simulink model "exp11_5"  (R2020a)
settings: Solver=FixedStepAuto  StartTime=0.0  StopTime=5  FixedStep=0.01  RelTol=1e-3
libraries: fl_lib x39, nesl_utility x3
settings Model: Creator=Sing Ngai  LastModifiedBy=zengw

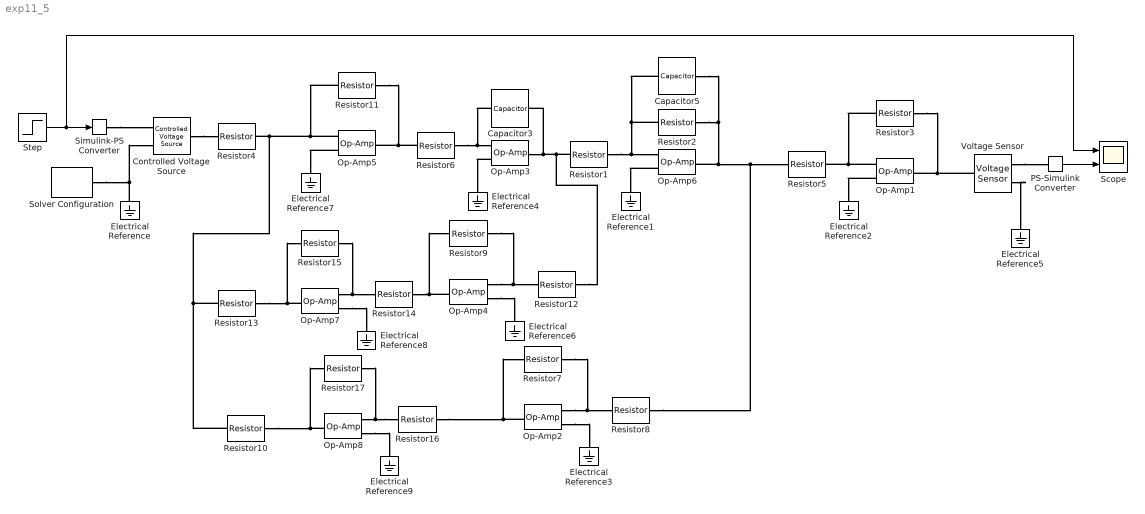
== system exp11_5 ==
  Capacitor3 : fl_lib/Electrical/Electrical Elements/Capacitor  c=2 uF  r=1e-6 Ohm  g=0 1/Ohm  i_specify=off  i_priority=None  i=0 A  i_nominal_specify=off  i_nominal_unit=A  i_nominal_value=1  v_specify=off  v_priority=None  v=0 V  v_nominal_specify=off  v_nominal_unit=V  v_nominal_value=1  vc_specify=off  vc_priority=High  vc=0 V  vc_nominal_specify=off  vc_nominal_unit=V  vc_nominal_value=1
  Capacitor5 : fl_lib/Electrical/Electrical Elements/Capacitor  c=1 uF  r=1e-6 Ohm  g=0 1/Ohm  i_specify=off  i_priority=None  i=0 A  i_nominal_specify=off  i_nominal_unit=A  i_nominal_value=1  v_specify=off  v_priority=None  v=0 V  v_nominal_specify=off  v_nominal_unit=V  v_nominal_value=1  vc_specify=off  vc_priority=High  vc=0 V  vc_nominal_specify=off  vc_nominal_unit=V  vc_nominal_value=1
  Controlled Voltage Source : fl_lib/Electrical/Electrical Sources/Controlled Voltage Source
  Electrical Reference{,1..9} (10 alike) : fl_lib/Electrical/Electrical Elements/Electrical Reference
  Op-Amp{1..8} (8 alike) : fl_lib/Electrical/Electrical Elements/Op-Amp  outI_specify=off  outI_priority=None  outI=0 A  outI_nominal_specify=off  outI_nominal_unit=A  outI_nominal_value=1
  PS-Simulink Converter : nesl_utility/PS-Simulink Converter  PhysicalDomain=network_engine_domain  SubClassName=ps_output  LeftPortType=input  RightPortType=output  PseudoPeriodic=off  Frequencies=[]  Unit=inherit  AffineConversion=off
  Resistor1 : fl_lib/Electrical/Electrical Elements/Resistor  R=50 kOhm  i_specify=off  i_priority=None  i=0 A  i_nominal_specify=off  i_nominal_unit=A  i_nominal_value=1  v_specify=off  v_priority=None  v=0 V  v_nominal_specify=off  v_nominal_unit=V  v_nominal_value=1
  Resistor{4,10..11,13} (4 alike) : fl_lib/Electrical/Electrical Elements/Resistor  R=200 kOhm  i_specify=off  i_priority=None  i=0 A  i_nominal_specify=off  i_nominal_unit=A  i_nominal_value=1  v_specify=off  v_priority=None  v=0 V  v_nominal_specify=off  v_nominal_unit=V  v_nominal_value=1
  Resistor{3,8,12,14..17} (7 alike) : fl_lib/Electrical/Electrical Elements/Resistor  R=100 kOhm  i_specify=off  i_priority=None  i=0 A  i_nominal_specify=off  i_nominal_unit=A  i_nominal_value=1  v_specify=off  v_priority=None  v=0 V  v_nominal_specify=off  v_nominal_unit=V  v_nominal_value=1
  Resistor2 : fl_lib/Electrical/Electrical Elements/Resistor  R=50 kOhm  i_specify=off  i_priority=None  i=0 A  i_nominal_specify=off  i_nominal_unit=A  i_nominal_value=1  v_specify=off  v_priority=None  v=0 V  v_nominal_specify=off  v_nominal_unit=V  v_nominal_value=1
  Resistor5 : fl_lib/Electrical/Electrical Elements/Resistor  R=20 kOhm  i_specify=off  i_priority=None  i=0 A  i_nominal_specify=off  i_nominal_unit=A  i_nominal_value=1  v_specify=off  v_priority=None  v=0 V  v_nominal_specify=off  v_nominal_unit=V  v_nominal_value=1
  Resistor6 : fl_lib/Electrical/Electrical Elements/Resistor  R=500 kOhm  i_specify=off  i_priority=None  i=0 A  i_nominal_specify=off  i_nominal_unit=A  i_nominal_value=1  v_specify=off  v_priority=None  v=0 V  v_nominal_specify=off  v_nominal_unit=V  v_nominal_value=1
  Resistor7 : fl_lib/Electrical/Electrical Elements/Resistor  R=1300 kOhm  i_specify=off  i_priority=None  i=0 A  i_nominal_specify=off  i_nominal_unit=A  i_nominal_value=1  v_specify=off  v_priority=None  v=0 V  v_nominal_specify=off  v_nominal_unit=V  v_nominal_value=1
  Resistor9 : fl_lib/Electrical/Electrical Elements/Resistor  R=800 kOhm  i_specify=off  i_priority=None  i=0 A  i_nominal_specify=off  i_nominal_unit=A  i_nominal_value=1  v_specify=off  v_priority=None  v=0 V  v_nominal_specify=off  v_nominal_unit=V  v_nominal_value=1
  Scope : Scope  NumInputPorts=2
  Simulink-PS Converter : nesl_utility/Simulink-PS Converter  PhysicalDomain=network_engine_domain  SubClassName=ps_input  LeftPortType=input  RightPortType=output  PseudoPeriodic=off  Frequencies=[]  NoiseDistribution=none  NoiseParameters=[]  Unit=1  AffineConversion=off  FilteringAndDerivatives=provide  SimscapeFilterOrder=1  InputFilterTimeConstant=0.001  UdotUserProvided=0
  Solver Configuration : nesl_utility/Solver Configuration  PhysicalDomain=network_engine_domain  SubClassName=solver  LeftPortType=input  RightPortType=generic  Tones=[]  Harmonics=[]  SimulateNoise=off  Profile=off  UseLocalSampling=off  EnableSwitchedLinearOptims=on  FrequencyDomain=off  UseCCode=off  RelTol=0.001  AbsTol=1e-06  MinStep=1e-09  ToWorkspace=off  RevertToSquareIcSolve=off  NumHomotopyIterations=100  PhasorMode=off  PhasorModeNumHarmonics=1  DoDC=off  ResidualTolerance=1e-09  UseLocalSolver=off  LocalSolverChoice=NE_BACKWARD_EULER_ADVANCER  LocalSolverSampleTime=0.001  DoFixedCost=off  MaxNonlinIter=3  MaxModeIter=2  LinearAlgebra=auto  EquationFormulation=NE_TIME_EF  DelaysMemoryBudget=1024  AutomaticFiltering=on  FilteringTimeConstant=0.001  PartitionStorageMethod=AS_NEEDED  PartitionMemoryBudget=1024  PartitionMethod=ROBUST
  Step : Step  Before=1  SampleTime=0
  Voltage Sensor : fl_lib/Electrical/Electrical Sensors/Voltage Sensor
  wires:
  Step/1 -> Scope/1, Simulink-PS Converter/1
  PS-Simulink Converter/1 -> Scope/2
  connections:
  Op-Amp6/RConn1 -- Resistor8/LConn1 -- Resistor5/LConn1 -- Capacitor5/RConn1 -- Resistor2/RConn1
  Solver Configuration/RConn1 -- Controlled Voltage Source/RConn2 -- Electrical Reference/LConn1
  Resistor1/RConn1 -- Op-Amp6/LConn2 -- Capacitor5/LConn1 -- Resistor2/LConn1
  Op-Amp7/RConn1 -- Resistor13/LConn1 -- Resistor15/RConn1
  Op-Amp1/LConn2 -- Resistor5/RConn1 -- Resistor3/LConn1
  Op-Amp5/RConn1 -- Resistor6/LConn1 -- Resistor11/RConn1
  Op-Amp1/RConn1 -- Voltage Sensor/LConn1 -- Resistor3/RConn1
  Capacitor3/LConn1 -- Op-Amp3/LConn2 -- Resistor6/RConn1
  Op-Amp3/RConn1 -- Resistor12/LConn1 -- Resistor1/LConn1 -- Capacitor3/RConn1
  Voltage Sensor/RConn2 -- Electrical Reference5/LConn1
  Voltage Sensor/RConn1 -- PS-Simulink Converter/LConn1
  Op-Amp5/LConn1 -- Electrical Reference7/LConn1
  Op-Amp1/LConn1 -- Electrical Reference2/LConn1
  Simulink-PS Converter/RConn1 -- Controlled Voltage Source/RConn1
  Op-Amp6/LConn1 -- Electrical Reference1/LConn1
  Controlled Voltage Source/LConn1 -- Resistor4/LConn1
  Op-Amp3/LConn1 -- Electrical Reference4/LConn1
  Op-Amp2/LConn2 -- Resistor8/RConn1 -- Resistor7/LConn1
  Op-Amp2/LConn1 -- Electrical Reference3/LConn1
  Op-Amp2/RConn1 -- Resistor7/RConn1 -- Resistor16/LConn1
  Op-Amp4/LConn2 -- Resistor12/RConn1 -- Resistor9/LConn1
  Op-Amp4/RConn1 -- Resistor14/LConn1 -- Resistor9/RConn1
  Op-Amp4/LConn1 -- Electrical Reference6/LConn1
  Op-Amp7/LConn2 -- Resistor15/LConn1 -- Resistor14/RConn1
  Op-Amp7/LConn1 -- Electrical Reference8/LConn1
  Resistor11/LConn1 -- Op-Amp5/LConn2 -- Resistor13/RConn1 -- Resistor10/LConn1 -- Resistor4/RConn1
  Op-Amp8/RConn1 -- Resistor17/RConn1 -- Resistor10/RConn1
  Resistor16/RConn1 -- Resistor17/LConn1 -- Op-Amp8/LConn2
  Op-Amp8/LConn1 -- Electrical Reference9/LConn1
